simulink model "phase_modul"  (R2020a)
settings: Solver=VariableStepAuto  StartTime=0.0  StopTime=010  MaxStep=.0001  RelTol=1e-3
settings Model: Creator=Atharv Sharma  LastModifiedBy=Atharv Sharma

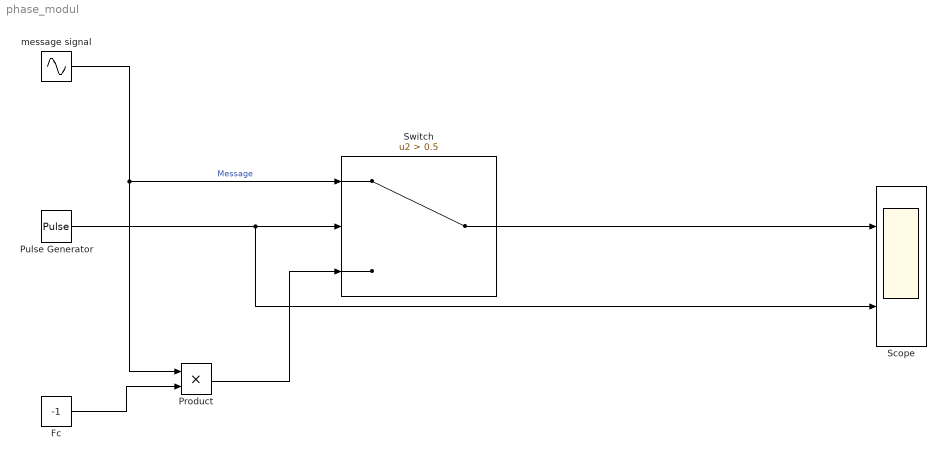
== system phase_modul ==
  Fc : Constant  Value=-1  SampleTime=.0001
  Product : Product
  Pulse Generator : DiscretePulseGenerator  PulseType=Time based  PulseWidth=50
  Scope : Scope  NumInputPorts=2
  Switch : Switch  Criteria=u2 > Threshold  Threshold=0.5
  message signal : Sin  Amplitude=20  Frequency=2*pi*2  SampleTime=.0001
  wires:
  Pulse Generator/1 -> Scope/2, Switch/2
  message signal/1 -> Product/1, Switch/1  "Message"
  Fc/1 -> Product/2
  Product/1 -> Switch/3
  Switch/1 -> Scope/1
